simulink model "DC_Charger"  (R2024b)
settings: Solver=ode23t  StartTime=0.0  StopTime=inf  FixedStep=1e-6  MaxStep=1/(5*inverter.SwitchFrequency)  RelTol=1e-3  AbsTol=1e-3
undefined symbols (not defined in the file or in its folder): battery, inverter, rectifier
libraries: nesl_utility x38, fl_lib x26, ee_lib x14, batteryecm_lib x3, eePwmGenerator x2, eeTransforms x2, eeSinusoidalMeasurement x1, slpidlib x1, eePwmGeneratorThreeLevel x1, eePwmGeneratorTwoLevel x1, simulink_extras x1
(part 1 of 3)
settings Model: Creator=The MathWorks, Inc.  LastModifiedBy=ganes
settings SolverCC: AutoScaleAbsTol=off  MaxZcPerStep=1
settings DataIOCC: SaveState=on  SignalLogging=off  DSMLogging=off  ReturnWorkspaceOutputs=off
settings OptimizationCC: ReuseModelBlockBuffer=off
settings DebuggingCC: IgnoredZcDiagnostic=none  UnconnectedInputMsg=warning  UnconnectedOutputMsg=warning  UnconnectedLineMsg=warning
settings ModelReferenceCC: EnableRefExpFcnMdlSchedulingChecks=on
settings RTWCC: GPUComputeCapability=3.5  DLArmComputeVersion=19.05
settings SimscapeCC: SimscapeLogType=all  SimscapeLogSimulationStatistics=on  SimscapeLogName=simlog_DCFastCharger  SimscapeLogLimitData=off

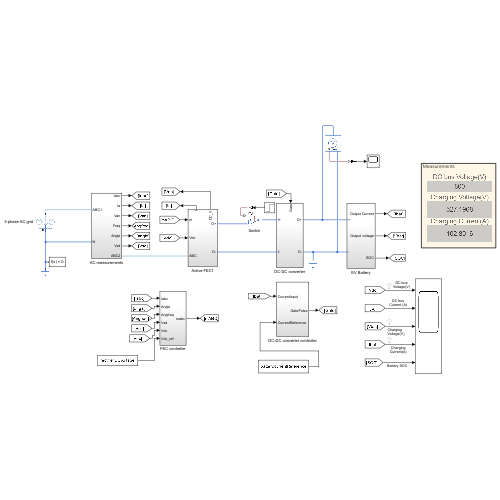
[thumbnail: Simulink's stored preview of the top-level diagram]
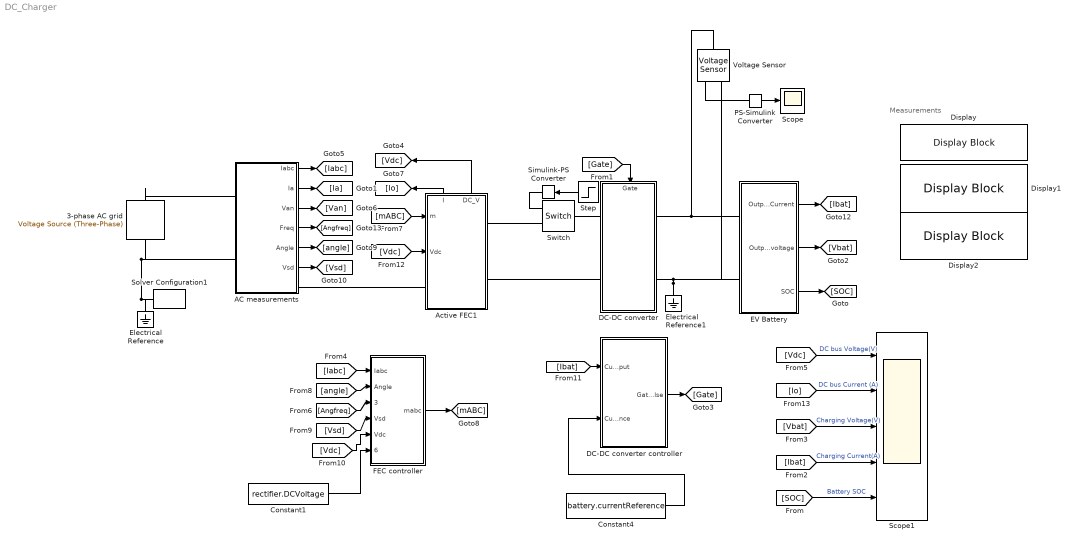
== system DC_Charger ==
  note: Measurements
  3-phase AC grid : ee_lib/Sources/Voltage Source (Three-Phase)  vline_rms=rectifier.ACVoltagePP V  shift=0 deg  freq=rectifier.SystemFrequency Hz  impedance_option=0  SShortCircuit=1e6 V*A  XR=15  R=0.01 Ohm  L=3.97e-4 H  harmonic_option=0  harmonic_orders=[5, 7, 11, 13]  harmonic_ratios=[.1, .1, .1, .1]  G_parasitic=0 1/Ohm  I_specify=off  I_priority=None  I=[ 0 0 0 ] A  I_nominal_specify=off  I_nominal_value=1  I_nominal_unit=A
  AC measurements : Subsystem
  Active FEC1 : Subsystem
      settings: PortSchema="{\"entries\":[{\"content\":{\"sides\":[{\"content\":{\"connectorIds\":[\"In1\",\"In2\",\"LConn1\"]},\"type\":\"ConnectorPlacement.EquallySpacedRectSide\",\"uuid\":\"e0050959-187d-4376-aad2-f8df21a08105\"},{\"content\":{\"connectorIds\":[\"RConn1\",\"RConn2\"],\"side\":\"RIGHT\"},\"type\":\"ConnectorPlacement.EquallySpacedRectSide\",\"uuid\":\"f7268924-358f-4021-b832-f47ce5e56f0e\"},{\"content\":{\"connectorIds\":[\"Out1\",\"Out2\"],\"side\":\"TOP\"},\"type\":\"ConnectorPlacement.EquallySpacedRectSide\",\"uuid\":\"ee33ccaf-ad48-493d-8220-739115e3c7e4\"}]},\"type\":\"ConnectorPlacement.EquallySpacedConnector\",\"uuid\":\"0bbfb8b2-bc26-491a-a2fb-5c6420aeb7c8\"}],\"packageUris\":[\"http://schema.mathworks.com/mf0/Connector/R2020b\"],\"version\":\"1.0\"}"
  Constant1 : Constant  Value=rectifier.DCVoltage
  Constant4 : Constant  Value=battery.currentReference
  DC-DC converter : Subsystem
      settings: PortSchema="{\"entries\":[{\"content\":{\"sides\":[{\"content\":{\"connectorIds\":[\"LConn1\",\"LConn2\"]},\"type\":\"ConnectorPlacement.EquallySpacedRectSide\",\"uuid\":\"cdc417bd-b70c-4a8b-af35-4387024a7132\"},{\"content\":{\"connectorIds\":[\"RConn1\",\"RConn2\"],\"side\":\"RIGHT\"},\"type\":\"ConnectorPlacement.EquallySpacedRectSide\",\"uuid\":\"7ffe8d7a-a957-4278-941d-227fd05ae124\"},{\"content\":{\"connectorIds\":[\"In1\"],\"side\":\"TOP\"},\"type\":\"ConnectorPlacement.EquallySpacedRectSide\",\"uuid\":\"a7a81929-1a7a-4c69-b225-a78f4f2fe477\"}]},\"type\":\"ConnectorPlacement.EquallySpacedConnector\",\"uuid\":\"ce8dd18f-fb87-4936-99a6-3d248ca5aaa5\"}],\"packageUris\":[\"http://schema.mathworks.com/mf0/Connector/R2020b\"],\"version\":\"1.0\"}"
  DC-DC converter controller : Subsystem
  Display : DisplayBlock  Format=Integer  Transparency=1  ShowGrid=off
  Display1 : DisplayBlock  Transparency=1
  Display2 : DisplayBlock  Transparency=1
  EV Battery : Subsystem
  Electrical Reference : fl_lib/Electrical/Electrical Elements/Electrical Reference
  Electrical Reference1 : fl_lib/Electrical/Electrical Elements/Electrical Reference
  FEC controller : Subsystem
  PS-Simulink Converter : nesl_utility/PS-Simulink Converter  PhysicalDomain=network_engine_domain  SubClassName=ps_output  LeftPortType=input  RightPortType=output  PseudoPeriodic=off  Frequencies=[]  VectorFormat=1-D array  Unit=inherit  AffineConversion=off
  Scope : Scope
  Scope1 : Scope  NumInputPorts=5
  Simulink-PS Converter : nesl_utility/Simulink-PS Converter  PhysicalDomain=network_engine_domain  SubClassName=ps_input  LeftPortType=input  RightPortType=output  PseudoPeriodic=off  Frequencies=[]  NoiseDistribution=none  NoiseParameters=[]  Unit=1  AffineConversion=off  FilteringAndDerivatives=provide  SimscapeFilterOrder=1  InputFilterTimeConstant=0.001  UdotUserProvided=0
  Solver Configuration1 : nesl_utility/Solver Configuration  PhysicalDomain=network_engine_domain  SubClassName=solver  LeftPortType=input  RightPortType=generic  Tones=[]  Harmonics=[]  SimulateNoise=off  Profile=off  UseLocalSampling=off  EnableSwitchedLinearOptims=on  FrequencyDomain=off  UseCCode=off  RelTol=0.001  AbsTol=1e-06  MinStep=1e-09  ToWorkspace=off  RevertToSquareIcSolve=off  NumHomotopyIterations=100  PhasorMode=off  PhasorModeNumHarmonics=1  ConsistencySolver=NEWTON_FTOL  IndexReductionMethod=DerivativeReplacement  DoDC=off  ResidualTolerance=1e-9  ConsistencyTolSource=GLOBAL  ConsistencyAbsTol=0.001  ConsistencyRelTol=0.001  ConsistencyTolFactor=0.001  UseLocalSolver=off  LocalSolverChoice=NE_PARTITIONING_ADVANCER  ResolveIndetEquations=on  FunctionEvalNumThread=1  LocalSolverSampleTime=1e-6  DoFixedCost=on  MaxNonlinIter=10  MaxModeIter=2  ComputeImpulses=off  ImpulseIterations=2  LinearAlgebra=auto  LinearAlgebraNumThread=0  EquationFormulation=NE_TIME_EF  DelaysMemoryBudget=1024  AutomaticFiltering=on  FilteringTimeConstant=0.001  PartitionStorageMethod=AS_NEEDED  PartitionMemoryBudget=1024  PartitionMethod=FAST  MultibodyUseLocalSolver=off  MultibodyLocalSolverChoice=ODE1  MultibodyLocalSolverSampleTime=0.001
  Step : Step  Time=0.02  SampleTime=0
  Switch : fl_lib/Electrical/Electrical Elements/Switch  R_closed=0.01 Ohm  G_open=1e-8 1/Ohm  Threshold=0.5  i_specify=off  i_priority=None  i=0 A  i_nominal_specify=off  i_nominal_value=1  i_nominal_unit=A  v_specify=off  v_priority=None  v=0 V  v_nominal_specify=off  v_nominal_value=1  v_nominal_unit=V
  Voltage Sensor : fl_lib/Electrical/Electrical Sensors/Voltage Sensor
  wires:
  [Gate] -> DC-DC converter/1(Gate)
  AC measurements/2(Ia) -> [Ia]
  [Angfreq] -> FEC controller/3(Angfreq)
  [Io] -> Scope1/2  "DC bus Current (A)"
  [angle] -> FEC controller/2(Angle)
  EV Battery/1(Output Current) -> [Ibat]
  PS-Simulink Converter/1 -> Scope/1
  [Vbat] -> Scope1/3  "Charging Voltage(V)"
  [SOC] -> Scope1/5  "Battery SOC"
  EV Battery/3(SOC) -> [SOC]
  AC measurements/3(Van) -> [Van]
  FEC controller/1(mabc) -> [mABC]
  [Ibat] -> DC-DC converter controller/1(CurrentInput)
  AC measurements/1(Iabc) -> [Iabc]
  [Vsd] -> FEC controller/4(Vsd)
  AC measurements/6(Vsd) -> [Vsd]
  Active FEC1/1(I) -> [Io]
  EV Battery/2(Output voltage) -> [Vbat]
  [Vdc] -> Active FEC1/2(Vdc)
  DC-DC converter controller/1(GatePulse) -> [Gate]
  Active FEC1/2(DC_V) -> [Vdc]
  [Vdc] -> FEC controller/5(Vdc)
  Step/1 -> Simulink-PS Converter/1
  Constant1/1 -> FEC controller/6(Vdc_ref)
  [Vdc] -> Scope1/1  "DC bus Voltage(V)"
  Constant4/1 -> DC-DC converter controller/2(CurrentReference)
  [mABC] -> Active FEC1/1(m)
  [Iabc] -> FEC controller/1(Iabc)
  AC measurements/5(Angle) -> [angle]
  AC measurements/4(Freq) -> [Angfreq]
  [Ibat] -> Scope1/4  "Charging Current(A)"
  connections:
  Electrical Reference1/LConn1 -- EV Battery/LConn2 -- Voltage Sensor/RConn2 -- DC-DC converter/RConn2
  Solver Configuration1/RConn1 -- Electrical Reference/LConn1 -- 3-phase AC grid/LConn1 -- AC measurements/LConn2
  Voltage Sensor/LConn1 -- DC-DC converter/RConn1 -- EV Battery/LConn1
  3-phase AC grid/RConn1 -- AC measurements/LConn1
  PS-Simulink Converter/LConn1 -- Voltage Sensor/RConn1
  Simulink-PS Converter/RConn1 -- Switch/RConn1
  Active FEC1/RConn1 -- Switch/RConn2
  Switch/LConn1 -- DC-DC converter/LConn1
  AC measurements/RConn1 -- Active FEC1/LConn1
  DC-DC converter/LConn2 -- Active FEC1/RConn2

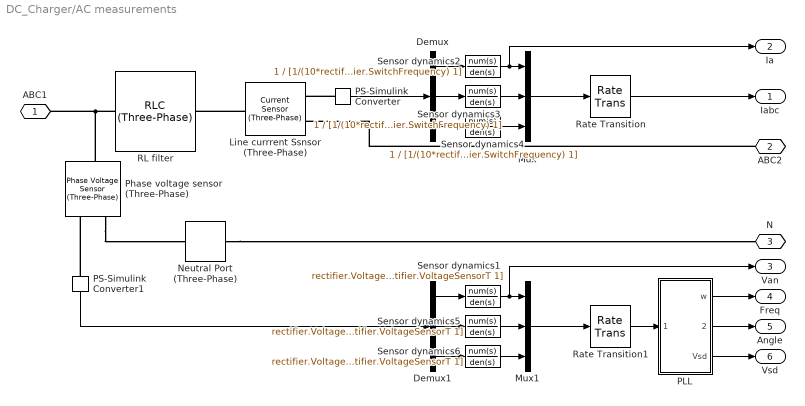
== system DC_Charger/AC measurements ==
  Demux : Demux  Outputs=3
  Demux1 : Demux  Outputs=3
  Line currrent Ssnsor (Three-Phase) : ee_lib/Sensors & Transducers/Current Sensor (Three-Phase)
  Mux : Mux  Inputs=3
  Mux1 : Mux  Inputs=3
  Neutral Port (Three-Phase) : ee_lib/Connectors & References/Neutral Port (Three-Phase)  G_parasitic=1e-12 1/Ohm
      settings: InternalSimscapePortConfiguration="{\"Bottom\":[],\"Left\":[{\"id\":\"N\",\"label\":\"~\",\"type\":\"foundation.electrical.three_phase\"}],\"Right\":[{\"id\":\"n\",\"label\":\"n\",\"type\":\"foundation.electrical.electrical\"}],\"Top\":[]}"
  PLL : Subsystem
  PS-Simulink Converter : nesl_utility/PS-Simulink Converter  PhysicalDomain=network_engine_domain  SubClassName=ps_output  LeftPortType=input  RightPortType=output  PseudoPeriodic=off  Frequencies=[]  VectorFormat=1-D array  Unit=inherit  AffineConversion=off
  PS-Simulink Converter1 : nesl_utility/PS-Simulink Converter  PhysicalDomain=network_engine_domain  SubClassName=ps_output  LeftPortType=input  RightPortType=output  PseudoPeriodic=off  Frequencies=[]  VectorFormat=1-D array  Unit=inherit  AffineConversion=off
  Phase voltage sensor (Three-Phase) : ee_lib/Sensors & Transducers/Phase Voltage Sensor (Three-Phase)
  RL filter : ee_lib/Passive/RLC Assemblies/RLC (Three-Phase)  port_option=ee.enum.threePhasePort.composite  component_structure=ee.enum.rlc.structure.SeriesRL  R=rectifier.lineResistance Ohm  L=rectifier.lineInductance H  C=1e-6 F  R_parasitic=1e-6 Ohm  G_parasitic=1e-6 1/Ohm  IL_specify=on  IL_priority=High  IL=[0, 0, 0] A  IL_nominal_specify=off  IL_nominal_value=1  IL_nominal_unit=A  VC_specify=on  VC_priority=High  VC=[0, 0, 0] V  VC_nominal_specify=off  VC_nominal_value=1  VC_nominal_unit=V
      settings: InternalSimscapePortConfiguration="{\"Bottom\":[],\"Left\":[{\"id\":\"N1\",\"label\":\"~1\",\"type\":\"foundation.electrical.three_phase\"}],\"Right\":[{\"id\":\"N2\",\"label\":\"~2\",\"type\":\"foundation.electrical.three_phase\"}],\"Top\":[]}"
  Rate Transition : RateTransition  OutPortSampleTime=1/(10*rectifier.SwitchFrequency)
  Rate Transition1 : RateTransition  OutPortSampleTime=rectifier.VoltageSensorT
  Sensor dynamics1 : TransferFcn  Numerator=rectifier.VoltageSensorG  Denominator=[rectifier.VoltageSensorT 1]
  Sensor dynamics2 : TransferFcn  Numerator=1  Denominator=[1/(10*rectifier.SwitchFrequency) 1]
  Sensor dynamics3 : TransferFcn  Numerator=1  Denominator=[1/(10*rectifier.SwitchFrequency) 1]
  Sensor dynamics4 : TransferFcn  Numerator=1  Denominator=[1/(10*rectifier.SwitchFrequency) 1]
  Sensor dynamics5 : TransferFcn  Numerator=rectifier.VoltageSensorG  Denominator=[rectifier.VoltageSensorT 1]
  Sensor dynamics6 : TransferFcn  Numerator=rectifier.VoltageSensorG  Denominator=[rectifier.VoltageSensorT 1]
  ABC1 : PMIOPort  Side=Left
  ABC2 : PMIOPort  Port=2  Side=Right
  N : PMIOPort  Port=3  Side=Left
  Iabc : Outport
  Ia : Outport  Port=2
  Van : Outport  Port=3
  Freq : Outport  Port=4
  Angle : Outport  Port=5
  Vsd : Outport  Port=6
  wires:
  Mux/1 -> Rate Transition/1
  Mux1/1 -> Rate Transition1/1
  PLL/3(Vsd) -> Vsd/1
  PLL/1(w) -> Freq/1
  PLL/2(angle) -> Angle/1
  Sensor dynamics4/1 -> Mux/3
  Demux/2 -> Sensor dynamics3/1
  Demux/3 -> Sensor dynamics4/1
  Demux/1 -> Sensor dynamics2/1
  Sensor dynamics2/1 -> Ia/1, Mux/1
  Sensor dynamics3/1 -> Mux/2
  Sensor dynamics6/1 -> Mux1/3
  Demux1/2 -> Sensor dynamics5/1
  Demux1/3 -> Sensor dynamics6/1
  Demux1/1 -> Sensor dynamics1/1
  Sensor dynamics1/1 -> Van/1, Mux1/1
  Sensor dynamics5/1 -> Mux1/2
  PS-Simulink Converter/1 -> Demux/1
  PS-Simulink Converter1/1 -> Demux1/1
  Rate Transition/1 -> Iabc/1
  Rate Transition1/1 -> PLL/1(Vabc)
  connections:
  Line currrent Ssnsor (Three-Phase)/LConn1 -- RL filter/RConn1
  ABC2/RConn1 -- Line currrent Ssnsor (Three-Phase)/RConn2
  PS-Simulink Converter/LConn1 -- Line currrent Ssnsor (Three-Phase)/RConn1
  PS-Simulink Converter1/LConn1 -- Phase voltage sensor (Three-Phase)/RConn1
  RL filter/LConn1 -- ABC1/RConn1 -- Phase voltage sensor (Three-Phase)/LConn1
  Neutral Port (Three-Phase)/RConn1 -- N/RConn1
  Phase voltage sensor (Three-Phase)/RConn2 -- Neutral Port (Three-Phase)/LConn1

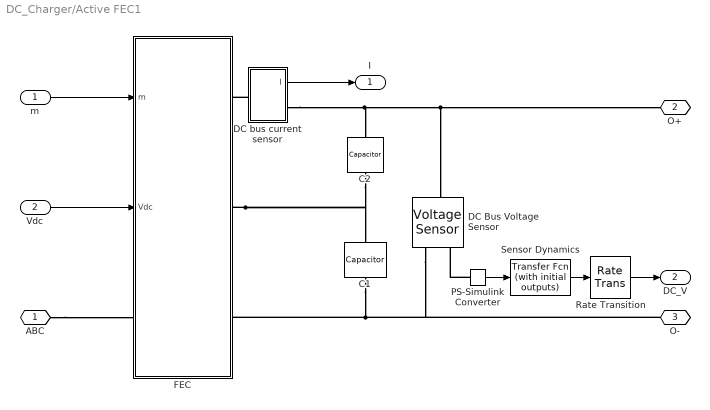
== system DC_Charger/Active FEC1 ==
  m : Inport
  Vdc : Inport  Port=2
  C1 : fl_lib/Electrical/Electrical Elements/Capacitor  c=rectifier.OutputCapacitance*2 F  r=0.1e-3 Ohm  g=0 1/Ohm  i_specify=off  i_priority=High  i=0 A  i_nominal_specify=off  i_nominal_value=1  i_nominal_unit=A  v_specify=off  v_priority=High  v=0 V  v_nominal_specify=off  v_nominal_value=1  v_nominal_unit=V  vc_specify=on  vc_priority=High  vc=(rectifier.ACVoltagePP*1.414)/2*1.5 V  vc_nominal_specify=off  vc_nominal_value=1  vc_nominal_unit=V
  C2 : fl_lib/Electrical/Electrical Elements/Capacitor  c=rectifier.OutputCapacitance*2 F  r=0.1e-3 Ohm  g=0 1/Ohm  i_specify=off  i_priority=High  i=0 A  i_nominal_specify=off  i_nominal_value=1  i_nominal_unit=A  v_specify=off  v_priority=High  v=0 V  v_nominal_specify=off  v_nominal_value=1  v_nominal_unit=V  vc_specify=on  vc_priority=High  vc=(rectifier.ACVoltagePP*1.414)/2*1.5 V  vc_nominal_specify=off  vc_nominal_value=1  vc_nominal_unit=V
  DC Bus Voltage Sensor : fl_lib/Electrical/Electrical Sensors/Voltage Sensor
  DC bus current sensor : Subsystem
  FEC : Subsystem  Variant=on  VariantControl=Variant1
  PS-Simulink Converter : nesl_utility/PS-Simulink Converter  PhysicalDomain=network_engine_domain  SubClassName=ps_output  LeftPortType=input  RightPortType=output  PseudoPeriodic=off  Frequencies=[]  VectorFormat=1-D array  Unit=inherit  AffineConversion=off
  Rate Transition : RateTransition  OutPortSampleTime=rectifier.VoltageSensorT
  Sensor Dynamics : simulink_extras/Additional Linear/Transfer Fcn (with initial outputs)  N=rectifier.VoltageSensorG  D=[rectifier.VoltageSensorT 1]  Y0=rectifier.ACVoltagePP*1.414  U0=rectifier.ACVoltagePP*1.414
  ABC : PMIOPort  Side=Left
  O+ : PMIOPort  Port=2  Side=Right
  O- : PMIOPort  Port=3  Side=Right
  I : Outport
  DC_V : Outport  Port=2
  wires:
  m/1 -> FEC/1(m)
  Vdc/1 -> FEC/2(Vdc)
  DC bus current sensor/1(I) -> I/1
  Sensor Dynamics/1 -> Rate Transition/1
  PS-Simulink Converter/1 -> Sensor Dynamics/1
  Rate Transition/1 -> DC_V/1
  connections:
  ABC/RConn1 -- FEC/LConn1
  C1/RConn1 -- O-/RConn1 -- DC Bus Voltage Sensor/RConn2 -- FEC/RConn3
  FEC/RConn2 -- C1/LConn1 -- C2/RConn1
  DC bus current sensor/LConn1 -- FEC/RConn1
  PS-Simulink Converter/LConn1 -- DC Bus Voltage Sensor/RConn1
  DC bus current sensor/RConn1 -- O+/RConn1 -- DC Bus Voltage Sensor/LConn1 -- C2/LConn1

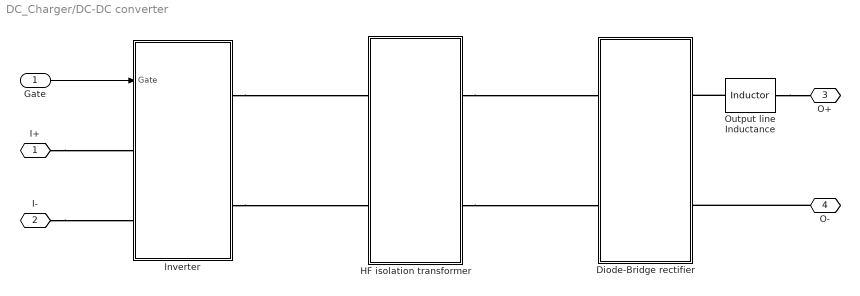
== system DC_Charger/DC-DC converter ==
  Gate : Inport
  Diode-Bridge rectifier : Subsystem
  HF isolation transformer : Subsystem
  Inverter : Subsystem
  Output line Inductance : ee_lib/Passive/Inductor  l=battery.inductance H  enable_L_tol=0  L_tol=20  tol_distribution=1  nSigma=4  r=0 Ohm  g=1e-9 1/Ohm  enable_operating_limits=0  operating_limit_action=2  max_working_current=1 A  power_rating=1 W  fault_action=simscape.enum.assert.action.none  t_fault=1 s  i_L_specify=off  i_L_priority=High  i_L=80 A  i_L_nominal_specify=off  i_L_nominal_value=1  i_L_nominal_unit=A
  I+ : PMIOPort  Side=Left
  I- : PMIOPort  Port=2  Side=Left
  O+ : PMIOPort  Port=3  Side=Right
  O- : PMIOPort  Port=4  Side=Right
  wires:
  Gate/1 -> Inverter/1(Gate)
  connections:
  Inverter/RConn2 -- HF isolation transformer/LConn2
  O-/RConn1 -- Diode-Bridge rectifier/RConn2
  Inverter/RConn1 -- HF isolation transformer/LConn1
  HF isolation transformer/RConn1 -- Diode-Bridge rectifier/LConn1
  HF isolation transformer/RConn2 -- Diode-Bridge rectifier/LConn2
  I+/RConn1 -- Inverter/LConn1
  I-/RConn1 -- Inverter/LConn2
  Output line Inductance/RConn1 -- O+/RConn1
  Output line Inductance/LConn1 -- Diode-Bridge rectifier/RConn1

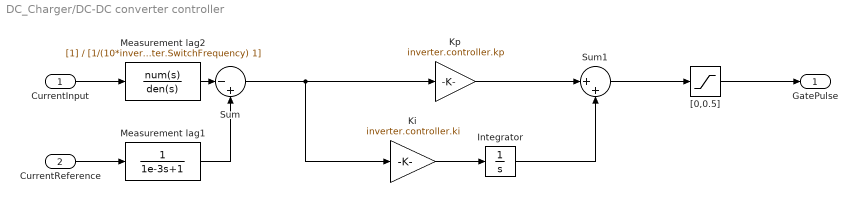
== system DC_Charger/DC-DC converter controller ==
  CurrentInput : Inport
  CurrentReference : Inport  Port=2
  Integrator : Integrator  LimitOutput=on  UpperSaturationLimit=3  LowerSaturationLimit=-3
  Ki : Gain  Gain=inverter.controller.ki
  Kp : Gain  Gain=inverter.controller.kp
  Measurement lag1 : TransferFcn  Denominator=[1e-3 1]
  Measurement lag2 : TransferFcn  Denominator=[1/(10*inverter.SwitchFrequency) 1]
  Sum : Sum  Inputs=|-+
  Sum1 : Sum  Inputs=|++  InputSameDT=on  SaturateOnIntegerOverflow=on  OutDataTypeStr=Inherit: Same as first input
  "[0,0.5]" : Saturate  LowerLimit=0
  GatePulse : Outport
  wires:
  Sum/1 -> Ki/1, Kp/1
  Sum1/1 -> "[0,0.5]"/1
  "[0,0.5]"/1 -> GatePulse/1
  Kp/1 -> Sum1/1
  Ki/1 -> Integrator/1
  Integrator/1 -> Sum1/2
  Measurement lag2/1 -> Sum/1
  Measurement lag1/1 -> Sum/2
  CurrentReference/1 -> Measurement lag1/1
  CurrentInput/1 -> Measurement lag2/1

== system DC_Charger/EV Battery ==
  EV Battery : Subsystem
      settings: PortSchema="{\"entries\":[{\"content\":{\"sides\":[{\"content\":{\"connectorIds\":[]},\"type\":\"ConnectorPlacement.EquallySpacedRectSide\",\"uuid\":\"8e1978f5-f19b-407a-84fd-c941bccecdad\"},{\"content\":{\"connectorIds\":[],\"side\":\"RIGHT\"},\"type\":\"ConnectorPlacement.EquallySpacedRectSide\",\"uuid\":\"fb49f29d-d34c-48f8-a58f-9f92c5d477c5\"},{\"content\":{\"connectorIds\":[\"LConn1\"],\"side\":\"TOP\"},\"type\":\"ConnectorPlacement.EquallySpacedRectSide\",\"uuid\":\"6762467a-e296-4691-a6dd-75c21ebdcdad\"},{\"content\":{\"connectorIds\":[\"Out1\",\"RConn1\"],\"side\":\"BOTTOM\"},\"type\":\"ConnectorPlacement.EquallySpacedRectSide\",\"uuid\":\"82209aad-7084-4f05-b357-bb8919115a4c\"}]},\"type\":\"ConnectorPlacement.EquallySpacedConnector\",\"uuid\":\"7c4645ca-e004-4a10-a314-5de950045894\"}],\"packageUris\":[\"http://schema.mathworks.com/mf0/Connector/R2020b\"],\"version\":\"1.0\"}"
  i : Subsystem
  v : Subsystem
  + : PMIOPort  Side=Left
  - : PMIOPort  Port=2  Side=Left
  Output Current : Outport
  Output voltage : Outport  Port=2
  SOC : Outport  Port=3
  wires:
  i/1(I) -> Output Current/1  "DC"
  v/1(V) -> Output voltage/1  "V"
  EV Battery/1(SOC) -> SOC/1
  connections:
  i/LConn1 -- +/RConn1
  -/RConn1 -- v/LConn1 -- EV Battery/RConn1
  i/RConn1 -- EV Battery/LConn1 -- v/RConn1

== system DC_Charger/FEC controller ==
  Iabc : Inport
  Angle : Inport  Port=2
  Angfreq : Inport  Port=3
  Vsd : Inport  Port=4
  Vdc : Inport  Port=5
  Vdc_ref : Inport  Port=6
  Controller : Subsystem
  Modulation Signal : Subsystem
  mabc : Outport
  wires:
  Controller/1(Vd) -> Modulation Signal/1(Vd)
  Modulation Signal/1(mabc) -> mabc/1
  Controller/2(Vq) -> Modulation Signal/2(Vq)
  Vsd/1 -> Controller/4(Vsd)
  Iabc/1 -> Controller/1(Iabc)
  Vdc/1 -> Controller/5(Vdc)
  Angle/1 -> Modulation Signal/3(Angle), Controller/2(Angle)
  Angfreq/1 -> Controller/3(Angfreq)
  Vdc_ref/1 -> Controller/6(Vdc_ref)

== system DC_Charger/AC measurements/PLL ==
  Vabc : Inport
  Constant : Constant  Value=pi/2
  Gain2 : Gain  Gain=2*pi
  "Sinusoidal measurement (PLL, Three-Phase)" : eeSinusoidalMeasurement/Sinusoidal Measurement (PLL, Three-Phase)  Kp_LF=0.05  Ki_LF=1  F0=rectifier.SystemFrequency  Theta0=0  Ts=rectifier.VoltageSensorT
  Subtract : Sum  Inputs=-+
  Vphm to Vsd : Gain  Gain=3/2
  w : Outport  VectorParamsAs1DForOutWhenUnconnected=off
  angle : Outport  Port=2  VectorParamsAs1DForOutWhenUnconnected=off
  Vsd : Outport  Port=3  VectorParamsAs1DForOutWhenUnconnected=off
  wires:
  "Sinusoidal measurement (PLL, Three-Phase)"/3 -> Vphm to Vsd/1
  Gain2/1 -> w/1
  "Sinusoidal measurement (PLL, Three-Phase)"/1 -> Gain2/1
  Vabc/1 -> "Sinusoidal measurement (PLL, Three-Phase)"/1
  Subtract/1 -> angle/1
  "Sinusoidal measurement (PLL, Three-Phase)"/2 -> Subtract/2
  Constant/1 -> Subtract/1
  Vphm to Vsd/1 -> Vsd/1

== system DC_Charger/Active FEC1/DC bus current sensor ==
  Current Sensor : fl_lib/Electrical/Electrical Sensors/Current Sensor
      settings: LogSimulationData=on
  PS-Simulink Converter1 : nesl_utility/PS-Simulink Converter  PhysicalDomain=network_engine_domain  SubClassName=ps_output  LeftPortType=input  RightPortType=output  PseudoPeriodic=off  Frequencies=[]  VectorFormat=1-D array  Unit=1  AffineConversion=off
  Sensor dynamics : TransferFcn  Numerator=1  Denominator=[1/(10*rectifier.SwitchFrequency) 1]
  + : PMIOPort  Side=Left
  - : PMIOPort  Port=2  Side=Right
  I : Outport
  wires:
  PS-Simulink Converter1/1 -> Sensor dynamics/1
  Sensor dynamics/1 -> I/1
  connections:
  Current Sensor/LConn1 -- +/RConn1
  PS-Simulink Converter1/LConn1 -- Current Sensor/RConn1
  Current Sensor/RConn2 -- -/RConn1

== system DC_Charger/Active FEC1/FEC ==
  m : Inport
  Vdc : Inport  Port=2
  Average : Subsystem  VariantControl=powerCircuit==0
  Three Level : Subsystem  VariantControl=powerCircuit==2
  Two Level : Subsystem  VariantControl=powerCircuit==1
  + : PMIOPort  Side=Right
  O : PMIOPort  Port=2  Side=Right
  - : PMIOPort  Port=3  Side=Right
  ABC : PMIOPort  Port=4  Side=Left

== system DC_Charger/DC-DC converter/Diode-Bridge rectifier ==
  Diode{1..4} (4 alike) : fl_lib/Electrical/Electrical Elements/Diode  Vf=0.6 V  Ron=0.01 Ohm  Goff=1e-8 1/Ohm  i_specify=off  i_priority=None  i=0 A  i_nominal_specify=off  i_nominal_value=1  i_nominal_unit=A  v_specify=off  v_priority=None  v=0 V  v_nominal_specify=off  v_nominal_value=1  v_nominal_unit=V
  + : PMIOPort  Side=Right
  P : PMIOPort  Port=2  Side=Left
  - : PMIOPort  Port=3  Side=Right
  N : PMIOPort  Port=4  Side=Left
  connections:
  Diode4/RConn1 -- Diode2/RConn1 -- +/RConn1
  Diode1/LConn1 -- Diode3/LConn1 -- -/RConn1
  Diode4/LConn1 -- Diode1/RConn1 -- P/RConn1
  Diode3/RConn1 -- N/RConn1 -- Diode2/LConn1

== system DC_Charger/DC-DC converter/HF isolation transformer ==
  Ideal Transformer : fl_lib/Electrical/Electrical Elements/Ideal Transformer  n=transformer.windingFactor  i1_specify=off  i1_priority=None  i1=0 A  i1_nominal_specify=off  i1_nominal_value=1  i1_nominal_unit=A  v1_specify=off  v1_priority=None  v1=0 V  v1_nominal_specify=off  v1_nominal_value=1  v1_nominal_unit=V  i2_specify=off  i2_priority=None  i2=0 A  i2_nominal_specify=off  i2_nominal_value=1  i2_nominal_unit=A  v2_specify=off  v2_priority=None  v2=0 V  v2_nominal_specify=off  v2_nominal_value=1  v2_nominal_unit=V
  Magnetizing Inductance : ee_lib/Passive/Inductor  l=transformer.magnetizingL H  enable_L_tol=0  L_tol=20  tol_distribution=1  nSigma=4  r=0 Ohm  g=1e-9 1/Ohm  enable_operating_limits=0  operating_limit_action=2  max_working_current=1 A  power_rating=1 W  fault_action=simscape.enum.assert.action.none  t_fault=1 s  i_L_specify=off  i_L_priority=High  i_L=0 A  i_L_nominal_specify=off  i_L_nominal_value=1  i_L_nominal_unit=A
  1+ : PMIOPort  Side=Left
  1- : PMIOPort  Port=2  Side=Left
  2+ : PMIOPort  Port=3  Side=Right
  2- : PMIOPort  Port=4  Side=Right
  connections:
  Ideal Transformer/RConn2 -- 2-/RConn1
  Ideal Transformer/LConn2 -- Magnetizing Inductance/RConn1 -- 1-/RConn1
  Ideal Transformer/LConn1 -- 1+/RConn1 -- Magnetizing Inductance/LConn1
  Ideal Transformer/RConn1 -- 2+/RConn1

== system DC_Charger/DC-DC converter/Inverter ==
  Gate : Inport
  Four-Quadrant Chopper : ee_lib/Semiconductors & Converters/Converters/Four-Quadrant Chopper  fidelity_option=ee.enum.converters.fidelity.detailed  device_type=ee.enum.converters.switchingdevice.ideal  showThermalPort=false  Vgt=1 V  Vgt_off=-1 V  Ih=1 A  Vf=0.8 V  Ron=0.001 Ohm  Rds=0.001 Ohm  Goff=1e-5 1/Ohm  Vth=0.8 V  K=0  Eon_scalar=22.86e-3 J  Eoff_scalar=17.14e-3 J  Eoff_natural_commutation=10e-3 J  Voff=300 V  Iout_scalar=600 A  onCurrentMeasDelay=0 s  useCurrentFromPreviousCycle=false  useVoltageFromPreviousCycle=false  diode_param=ee.enum.converters.protectiondiode.nodynamics  diode_Vf=0.8 V  diode_Ron=0.001 Ohm  diode_Goff=1e-5 1/Ohm  diode_C=50 nF  diode_iRM=-235 A  diode_iF=300 A  diode_idot=-50 A/us  diode_trr_param=ee.enum.converters.diodetrr.trr_factor  diode_trr_factor=3  diode_trr=15 us  diode_Qrr=1500 s*uA  diode_rec_loss_model=ee.enum.diode.reverseRecoveryModel.fixed  diode_ErecVal=0 J  diode_scaleWithIandV=false  diode_ErecMat=zeros(2, 3) J  diode_TjrecVec=[298.15, 398.15] K  diode_IfrecVec=[.1, 1, 10] A  diode_IrecVal=10 A  diode_VrecVal=10 V  diode_tFilter=1 / 1000 / 100 s  thermal_network_parameterization=ee.enum.thermalNetworkTopology.external  Rth=[.08, .5] K/W  Rth_Cauer=[.08, .1, .5] K/W  Rth_Foster=[.08, .14, .22, .16] K/W  thermal_mass_parameterization=ee.enum.thermalNetwork.timeconstant  thermal_mass=[.01, .5] J/K  thermal_mass_Cauer=[.01, .1, .5] J/K  thermal_mass_Foster=[.001, .005, .05, .5] J/K  thermal_time_constant=[.001, .2] s  thermal_time_constant_Cauer=[.001, .1, .2] s  thermal_time_constant_Foster=[7e-05, .0007, .01, .08] s  thermal_mass_initial_temperatures=[25, 25] degC  thermal_mass_initial_temperatures_Cauer=[25, 25, 25] degC  junction_thermal_mass=0.01 J/K  Tvec_initial_Foster=[25, 25, 25, 25] degC  snubber_type=ee.enum.converters.snubber.exclude  Cs=1e-7 F  Rs=0.1 Ohm
      settings: InternalSimscapePortConfiguration="{\"Bottom\":[],\"Left\":[{\"id\":\"G\",\"label\":\"G\",\"type\":\"foundation.electrical.eight_phase\"},{\"id\":\"p1\",\"label\":\"1+\",\"type\":\"foundation.electrical.electrical\"},{\"id\":\"n1\",\"label\":\"1-\",\"type\":\"foundation.electrical.electrical\"}],\"Right\":[{\"id\":\"p2\",\"label\":\"2+\",\"type\":\"foundation.electrical.electrical\"},{\"id\":\"n2\",\"label\":\"2-\",\"type\":\"foundation.electrical.electrical\"}],\"Top\":[]}"
  Gate drive : Subsystem
  P : PMIOPort  Side=Right
  + : PMIOPort  Port=2  Side=Left
  N : PMIOPort  Port=3  Side=Right
  - : PMIOPort  Port=4  Side=Left
  wires:
  Gate/1 -> Gate drive/1(Gate)
  connections:
  -/RConn1 -- Four-Quadrant Chopper/LConn3
  +/RConn1 -- Four-Quadrant Chopper/LConn2
  P/RConn1 -- Four-Quadrant Chopper/RConn1
  Four-Quadrant Chopper/RConn2 -- N/RConn1
  Gate drive/RConn1 -- Four-Quadrant Chopper/LConn1
